simulink model "P414_1_model02"  (R2021a)
settings: Solver=VariableStepAuto  StartTime=0.0  StopTime=1  RelTol=1e-3
values from neighbouring files (symbols this model uses):
  crop__C = [0.01 0.001 0.01 0.01]    [params.mat]
  crop__N = [0 0 0 0 0 0 0 0]    [params.mat]
  crop__R = [0 0 0]    [params.mat]
  heater__T = 288    [params.mat]
  subtrate__N = [1e-06 1e-06 1e-06 1e-06 1e-06 1e-06 1e-06 1e-06]    [params.mat]
  Tmax = 296    [P414_1_script.m]    (also in params.mat)
  Tstart = 285.5    [P414_1_script.m]    (also in params.mat)
libraries: HORTISIM x15
settings Model: VariantFading=off  Creator=djoroya  LastModifiedBy=djoroya
settings SolverCC: MaxConsecutiveMinStep=2
settings HardwareCC: TargetBitPerLong=64  TargetBitPerPointer=64  TargetBitPerSizeT=64  TargetBitPerPtrDiffT=64  TargetLongLongMode=on  TargetIntDivRoundTo=Zero  TargetEndianess=LittleEndian  TargetWordSize=64  TargetHWDeviceType=MATLAB Host  ProdEqTarget=off
settings RTWCC: Description=Rapid Simulation Target  SystemTargetFile=rsim.tlc  TemplateMakefile=rsim_default_tmf
settings RSimTargetCC: TargetLangStandard=C99 (ISO)

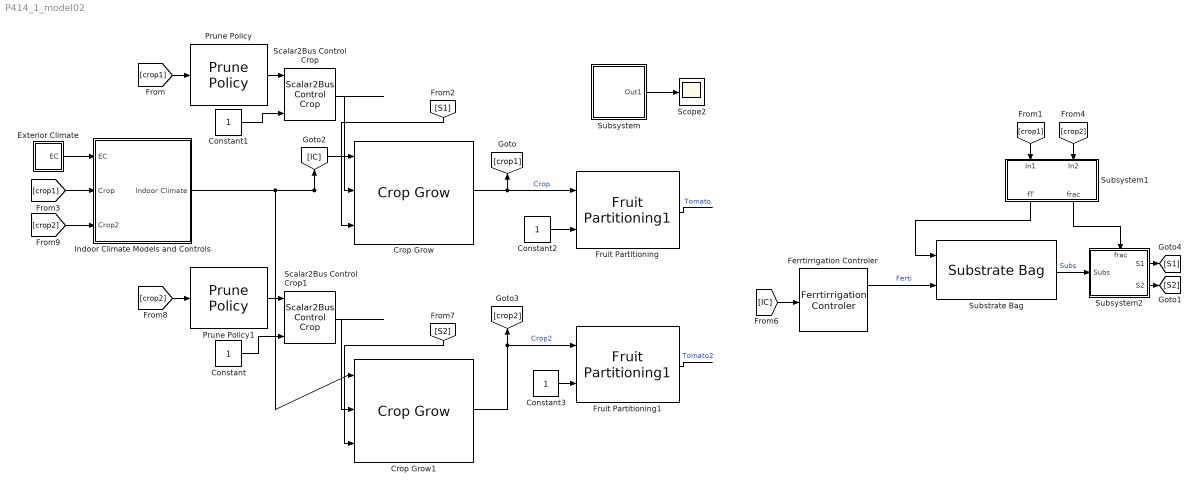
== system P414_1_model02 ==
  Constant{,1..3} (4 alike) : Constant
  Crop Grow : HORTISIM/Horticulture/Models/Crop Grow  Chi_nutrients=crop__Chi_nutrients  A_v=crop__A_v  plants_density=crop__plants_density  fraction_DM=crop__fraction_DM  min_water_capacity=crop__min_water_capacity  C_buf_max=crop__C_buf_max  T_v_start_fruit=crop__T_v_start_fruit  int_air_speed=crop__int_air_speed  b_N_uptake=crop__b_N_uptake  Tv=crop__Tv  C=crop__C  R=crop__R  Tsum=crop__Tsum  C_wv=crop__C_wv  N=crop__N  rg_fruit=crop__rg_fruit  c_fruit_m=crop__c_fruit_m  c_fruit_g=crop__c_fruit_g  rg_leaf=crop__rg_leaf  c_leaf_m=crop__c_leaf_m  c_leaf_g=crop__c_leaf_g  rg_stem=crop__rg_stem  c_stem_m=crop__c_stem_m  c_stem_g=crop__c_stem_g  VelocityAbsortion=crop__VelocityAbsortion  T_max_v=crop__T_max_v  s_max_T=crop__s_max_T  s_min_T=crop__s_min_T  s_buforg_buf=crop__s_buforg_buf  T_sum_end=crop__T_sum_end  T_max_v24=crop__T_max_v24  T_min_v24=crop__T_min_v24  s_min_T24=crop__s_min_T24  s_max_T24=crop__s_max_T24  T_min_v=crop__T_min_v
      settings: SourceProductName=Horti Simulator
  Crop Grow1 : HORTISIM/Horticulture/Models/Crop Grow  Chi_nutrients=crop__Chi_nutrients  A_v=crop__A_v  plants_density=crop__plants_density  fraction_DM=crop__fraction_DM  min_water_capacity=crop__min_water_capacity  C_buf_max=crop__C_buf_max  T_v_start_fruit=crop__T_v_start_fruit  int_air_speed=crop__int_air_speed  b_N_uptake=crop__b_N_uptake  Tv=crop__Tv  C=crop__C  R=crop__R  Tsum=crop__Tsum  C_wv=crop__C_wv  N=crop__N  rg_fruit=crop__rg_fruit  c_fruit_m=crop__c_fruit_m  c_fruit_g=crop__c_fruit_g  rg_leaf=crop__rg_leaf  c_leaf_m=crop__c_leaf_m  c_leaf_g=crop__c_leaf_g  rg_stem=crop__rg_stem  c_stem_m=crop__c_stem_m  c_stem_g=crop__c_stem_g  VelocityAbsortion=crop__VelocityAbsortion  T_max_v=crop__T_max_v  s_max_T=crop__s_max_T  s_min_T=crop__s_min_T  s_buforg_buf=crop__s_buforg_buf  T_sum_end=crop__T_sum_end  T_max_v24=crop__T_max_v24  T_min_v24=crop__T_min_v24  s_min_T24=crop__s_min_T24  s_max_T24=crop__s_max_T24  T_min_v=crop__T_min_v
      settings: SourceProductName=Horti Simulator
  Exterior Climate : Subsystem
  Ferrtirrigation Controler : HORTISIM/Horticulture/Controls/Ferrtirrigation  Controler  hour0=irrigation__hour0  IrrigationFlow=irrigation__IrrigationFlow  Xnutrients=irrigation__Xnutrients  percent_irrigation=irrigation__percent_irrigation  Irrigation_jules_to_hours=irrigation__Irrigation_jules_to_hours
      settings: SourceProductName=Horti Simulator
  Fruit Partitioning : HORTISIM/Horticulture/Models/Fruit Partitioning1  Cfruit0=tomato__Cfruit0
      settings: SourceProductName=Horti Simulator
  Fruit Partitioning1 : HORTISIM/Horticulture/Models/Fruit Partitioning1  Cfruit0=tomato__Cfruit0
      settings: SourceProductName=Horti Simulator
  Indoor Climate Models and Controls : Subsystem
  Prune Policy : HORTISIM/Horticulture/Controls/Prune Policy  SystemSampleTime=-1  VariantActivationTime=update diagram  Latency=0  AutoFrameSizeCalculation=off
      settings: SourceProductName=Horti Simulator
  Prune Policy1 : HORTISIM/Horticulture/Controls/Prune Policy  SystemSampleTime=-1  VariantActivationTime=update diagram  Latency=0  AutoFrameSizeCalculation=off
      settings: SourceProductName=Horti Simulator
  Scalar2Bus Control Crop : HORTISIM/Other  Functions/Scalar2Bus Control Crop  SystemSampleTime=-1  VariantActivationTime=update diagram  Latency=0  AutoFrameSizeCalculation=off
      settings: SourceProductName=Horti Simulator
  Scalar2Bus Control Crop1 : HORTISIM/Other  Functions/Scalar2Bus Control Crop  SystemSampleTime=-1  VariantActivationTime=update diagram  Latency=0  AutoFrameSizeCalculation=off
      settings: SourceProductName=Horti Simulator
  Scope2 : Scope
  Substrate Bag : HORTISIM/Horticulture/Models/Substrate Bag  Vmax_subs=subtrate__Vmax_subs  Vmin_subs=subtrate__Vmin_subs  Nmin_subs=subtrate__Nmin_subs  C_ws=subtrate__C_ws  N=subtrate__N  DraingeConst=subtrate__DraingeConst  sigma_max=subtrate__sigma_max  sigma_min=subtrate__sigma_min
      settings: SourceProductName=Horti Simulator
  Subsystem : Subsystem  mask{tinit=0.5, tend=0.8}
  Subsystem1 : Subsystem
  Subsystem2 : Subsystem
      settings: PortSchema="{\"entries\":[{\"content\":{\"sides\":[{\"content\":{\"connectorIds\":[\"In1\"]},\"type\":\"ConnectorPlacement.EquallySpacedRectSide\",\"uuid\":\"526c2ba0-7984-4a67-b75e-815cf79b4473\"},{\"content\":{\"connectorIds\":[\"Out1\",\"Out2\"],\"side\":\"RIGHT\"},\"type\":\"ConnectorPlacement.EquallySpacedRectSide\",\"uuid\":\"1f428ce7-4be7-4b4c-9b6b-ebbf12a2ebe7\"},{\"content\":{\"connectorIds\":[\"In2\"],\"side\":\"TOP\"},\"type\":\"ConnectorPlacement.EquallySpacedRectSide\",\"uuid\":\"5866ee80-50d2-4205-943e-212db577b0a0\"}]},\"type\":\"ConnectorPlacement.EquallySpacedConnector\",\"uuid\":\"0f7aadc1-005b-462a-894f-416c66164dac\"}],\"packageUris\":[\"http://schema.mathworks.com/mf0/Connector/R2020b\"],\"version\":\"1.0\"}"
  wires:
  Exterior Climate/1(EC) -> Indoor Climate Models and Controls/1(EC)
  Indoor Climate Models and Controls/1(Indoor Climate) -> Crop Grow1/1, [IC], Crop Grow/1
  Crop Grow/1 -> [crop1], Fruit Partitioning/1  "Crop"
  Ferrtirrigation Controler/1 -> Substrate Bag/2  "Ferti"
  Scalar2Bus Control Crop/1 -> Crop Grow/2
  Prune Policy/1 -> Scalar2Bus Control Crop/1
  [crop1] -> Prune Policy/1
  [S1] -> Crop Grow/3
  [crop1] -> Indoor Climate Models and Controls/2(Crop)
  Fruit Partitioning/1 -> ?  "Tomato"
  [IC] -> Ferrtirrigation Controler/1
  Crop Grow1/1 -> [crop2], Fruit Partitioning1/1  "Crop2"
  Fruit Partitioning1/1 -> ?  "Tomato2"
  Subsystem/1(Out1) -> Scope2/1
  [S2] -> Crop Grow1/3
  [crop2] -> Prune Policy1/1
  Scalar2Bus Control Crop1/1 -> Crop Grow1/2
  Prune Policy1/1 -> Scalar2Bus Control Crop1/1
  Constant/1 -> Scalar2Bus Control Crop1/4
  Constant1/1 -> Scalar2Bus Control Crop/4
  Constant2/1 -> Fruit Partitioning/2
  Constant3/1 -> Fruit Partitioning1/2
  [crop2] -> Indoor Climate Models and Controls/3(Crop2)
  [crop1] -> Subsystem1/1(In1)
  [crop2] -> Subsystem1/2(In2)
  Subsystem1/1(fT) -> Substrate Bag/1
  Substrate Bag/1 -> Subsystem2/1(Subs)  "Subs"
  Subsystem1/2(frac) -> Subsystem2/2(frac)
  Subsystem2/2(S2) -> [S2]
  Subsystem2/1(S1) -> [S1]

== system P414_1_model02/Exterior Climate ==
  Demux : Demux
  From Workspace : FromWorkspace  VariableName=EC
  Scalar2Bus Exterior Climate : Subsystem
  EC : Outport
  wires:
  Demux/3 -> Scalar2Bus Exterior Climate/3(Wind)
  Demux/2 -> Scalar2Bus Exterior Climate/2(Radiation)
  Scalar2Bus Exterior Climate/1(EC) -> EC/1
  Demux/1 -> Scalar2Bus Exterior Climate/1(Temperature)
  Demux/4 -> Scalar2Bus Exterior Climate/4(Humidity)
  From Workspace/1 -> Demux/1

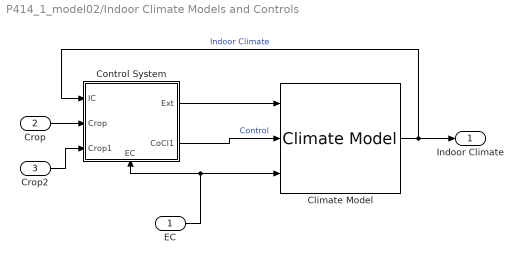
== system P414_1_model02/Indoor Climate Models and Controls ==
  EC : Inport
  Crop : Inport  Port=2
  Crop2 : Inport  Port=3
  Climate Model : HORTISIM/Climate/Models/Climate Model  hour0=clima__hour0  G0=clima__G0  T0=clima__T0  H=clima__H  A_f=clima__A_f  A_c=clima__A_c  minWindows=clima__minWindows  lam_s=clima__lam_s  c_s=clima__c_s  l_s=clima__l_s  rhod_s=clima__rhod_s  int_air_speed=clima__int_air_speed  alpha_i=clima__alpha_i  alpha_c=clima__alpha_c  tau_c=clima__tau_c  alpha_f=clima__alpha_f  d_c=clima__d_c  cd_c=clima__cd_c  T_ss=clima__T_ss
      settings: SourceProductName=Horti Simulator
  Control System : Subsystem
      settings: PortSchema="{\"entries\":[{\"content\":{\"sides\":[{\"content\":{\"connectorIds\":[\"In1\",\"In2\",\"In3\"]},\"type\":\"ConnectorPlacement.EquallySpacedRectSide\",\"uuid\":\"7d0146e2-a53b-49ab-a7f4-04cd7ef00b9a\"},{\"content\":{\"connectorIds\":[\"Out1\",\"Out2\"],\"side\":\"RIGHT\"},\"type\":\"ConnectorPlacement.EquallySpacedRectSide\",\"uuid\":\"fee587e2-4b5c-4140-8904-07609d427593\"},{\"content\":{\"connectorIds\":[],\"side\":\"TOP\"},\"type\":\"ConnectorPlacement.EquallySpacedRectSide\",\"uuid\":\"52e767bc-1595-40ac-996f-44c9eedd0a08\"},{\"content\":{\"connectorIds\":[\"In4\"],\"side\":\"BOTTOM\"},\"type\":\"ConnectorPlacement.EquallySpacedRectSide\",\"uuid\":\"c629db5c-cfe6-4bd1-aeb9-7fba46dde396\"}]},\"type\":\"ConnectorPlacement.EquallySpacedConnector\",\"uuid\":\"268fde01-3c08-4d62-bfbb-fc94284c5cdd\"}],\"packageUris\":[\"http://schema.mathworks.com/mf0/Connector/R2020b\"],\"version\":\"1.0\"}"
  Indoor Climate : Outport
  wires:
  Climate Model/1 -> Indoor Climate/1, Control System/1(IC)  "Indoor Climate"
  Control System/2(CoCl1) -> Climate Model/2  "Control"
  Control System/1(Ext) -> Climate Model/1
  EC/1 -> Control System/4(EC), Climate Model/3
  Crop/1 -> Control System/2(Crop)
  Crop2/1 -> Control System/3(Crop1)

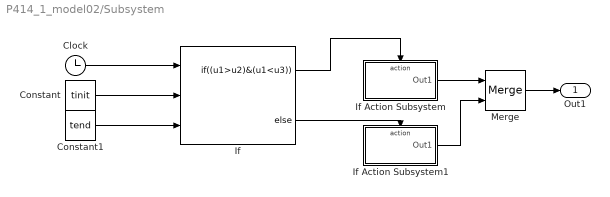
== system P414_1_model02/Subsystem ==
  Clock : Clock
  Constant : Constant  Value=tinit
  Constant1 : Constant  Value=tend
  If : If  NumInputs=3  IfExpression=(u1>u2)&(u1<u3)
  If Action Subsystem : Subsystem  TreatAsAtomicUnit=on
  If Action Subsystem1 : Subsystem  TreatAsAtomicUnit=on
  Merge : Merge
  Out1 : Outport
  wires:
  Clock/1 -> If/1
  Constant/1 -> If/2
  Constant1/1 -> If/3
  If/1 -> If Action Subsystem/Action
  If/2 -> If Action Subsystem1/Action
  If Action Subsystem/1(Out1) -> Merge/1
  If Action Subsystem1/1(Out1) -> Merge/2
  Merge/1 -> Out1/1

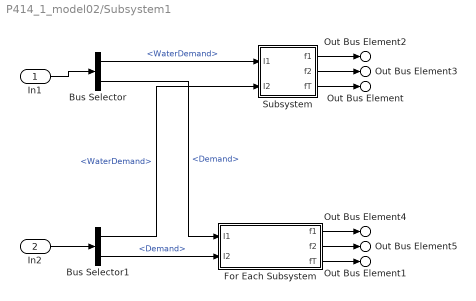
== system P414_1_model02/Subsystem1 ==
  In1 : Inport
  In2 : Inport  Port=2
  Bus Selector : BusSelector  OutputSignals=Water.WaterFlows.WaterDemand,Nutrients.Demand
  Bus Selector1 : BusSelector  OutputSignals=Water.WaterFlows.WaterDemand,Nutrients.Demand
  For Each Subsystem : Subsystem  TreatAsAtomicUnit=on
  Subsystem : Subsystem
  Out Bus Element1 : Outport  PortName=fT  Element=Nutrients.Demand
  Out Bus Element : Outport  PortName=fT  Element=Water.WaterFlows.WaterDemand
  Out Bus Element2 : Outport  Port=2  PortName=frac  Element=water.f1
  Out Bus Element3 : Outport  Port=2  PortName=frac  Element=water.f2
  Out Bus Element4 : Outport  Port=2  PortName=frac  Element=nutrients.f1
  Out Bus Element5 : Outport  Port=2  PortName=frac  Element=nutrients.f2
  wires:
  In1/1 -> Bus Selector/1
  In2/1 -> Bus Selector1/1
  Bus Selector1/1 -> Subsystem/2(I2)  "<WaterDemand>"
  Bus Selector/1 -> Subsystem/1(I1)  "<WaterDemand>"
  Subsystem/3(fT) -> Out Bus Element/1
  Subsystem/1(f1) -> Out Bus Element2/1
  Subsystem/2(f2) -> Out Bus Element3/1
  Bus Selector/2 -> For Each Subsystem/1(I1)  "<Demand>"
  Bus Selector1/2 -> For Each Subsystem/2(I2)  "<Demand>"
  For Each Subsystem/3(fT) -> Out Bus Element1/1
  For Each Subsystem/2(f2) -> Out Bus Element5/1
  For Each Subsystem/1(f1) -> Out Bus Element4/1

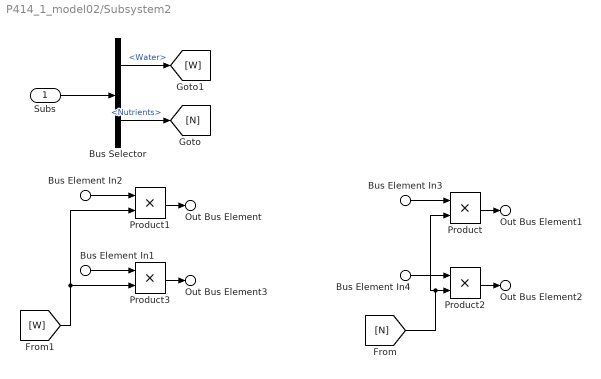
== system P414_1_model02/Subsystem2 ==
  Subs : Inport
  Bus Element In2 : Inport  Port=2  PortName=frac  Element=water.f1
  Bus Element In1 : Inport  Port=2  PortName=frac  Element=water.f2
  Bus Element In3 : Inport  Port=2  PortName=frac  Element=nutrients.f1
  Bus Element In4 : Inport  Port=2  PortName=frac  Element=nutrients.f2
  Bus Selector : BusSelector  OutputSignals=Uptake.Water,Uptake.Nutrients
  Product{,1..3} (4 alike) : Product
  Out Bus Element : Outport  PortName=S1  Element=Uptake.Water
  Out Bus Element1 : Outport  PortName=S1  Element=Uptake.Nutrients
  Out Bus Element3 : Outport  Port=2  PortName=S2  Element=Uptake.Water
  Out Bus Element2 : Outport  Port=2  PortName=S2  Element=Uptake.Nutrients
  wires:
  Subs/1 -> Bus Selector/1
  Bus Selector/1 -> [W]  "<Water>"
  Bus Selector/2 -> [N]  "<Nutrients>"
  Bus Element In3/1 -> Product/1
  Bus Element In2/1 -> Product1/1
  Bus Element In4/1 -> Product2/1
  [N] -> Product/2, Product2/2
  Bus Element In1/1 -> Product3/1
  [W] -> Product3/2, Product1/2
  Product1/1 -> Out Bus Element/1
  Product3/1 -> Out Bus Element3/1
  Product/1 -> Out Bus Element1/1
  Product2/1 -> Out Bus Element2/1

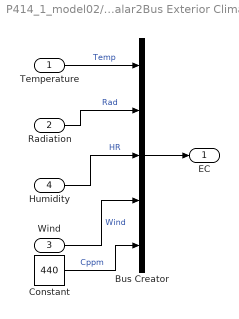
== system P414_1_model02/Exterior Climate/Scalar2Bus Exterior Climate ==
  Temperature : Inport
  Radiation : Inport  Port=2
  Wind : Inport  Port=3
  Humidity : Inport  Port=4
  Bus Creator : BusCreator  Inputs=5
  Constant : Constant  Value=440
  EC : Outport
  wires:
  Humidity/1 -> Bus Creator/3  "HR"
  Wind/1 -> Bus Creator/4  "Wind"
  Temperature/1 -> Bus Creator/1  "Temp"
  Bus Creator/1 -> EC/1
  Radiation/1 -> Bus Creator/2  "Rad"
  Constant/1 -> Bus Creator/5  "Cppm"

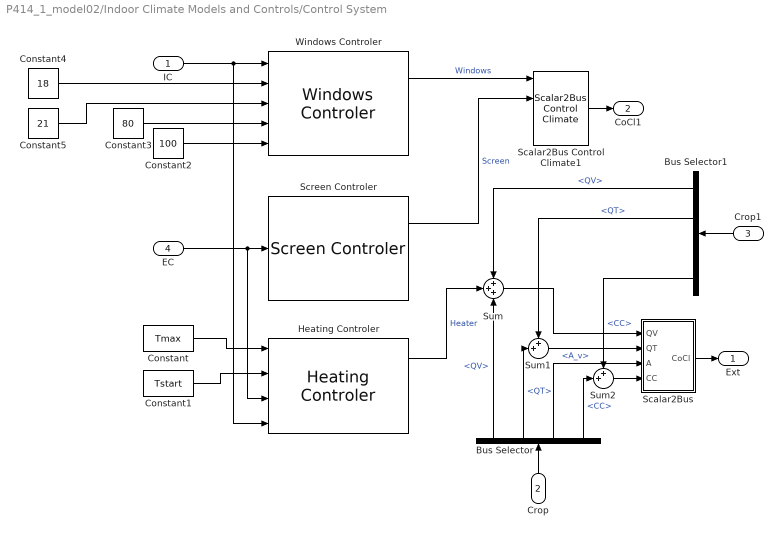
== system P414_1_model02/Indoor Climate Models and Controls/Control System ==
  IC : Inport
  Crop : Inport  Port=2
  Crop1 : Inport  Port=3
  EC : Inport  Port=4
  Bus Selector : BusSelector  OutputSignals=HeatVars.QV,HeatVars.QT,A_v,CC
  Bus Selector1 : BusSelector  OutputSignals=HeatVars.QV,HeatVars.QT,A_v,CC
  Constant : Constant  Value=Tmax
  Constant1 : Constant  Value=Tstart
  Constant2 : Constant  Value=100
  Constant3 : Constant  Value=80
  Constant4 : Constant  Value=18
  Constant5 : Constant  Value=21
  Heating Controler : HORTISIM/Climate/Controls/Heating Controler  T=heater__T  power=heater__power  A_e=heater__A_e  A_i=heater__A_i  c=heater__c
      settings: SourceProductName=Horti Simulator
  "Scalar2Bus " : Subsystem
  Scalar2Bus Control Climate1 : HORTISIM/Other  Functions/Scalar2Bus  Control Climate  SystemSampleTime=-1  VariantActivationTime=update diagram  Latency=0  AutoFrameSizeCalculation=off
      settings: SourceProductName=Horti Simulator
  Screen Controler : HORTISIM/Climate/Controls/Screen Controler  Radthreshold=screen__Radthreshold  velocity=screen__velocity  Power=screen__Power  gamma_max=screen__gamma_max  beta=screen__beta
      settings: SourceProductName=Horti Simulator
  Sum : Sum  Inputs=+++
  Sum1 : Sum  Inputs=++|
  Sum2 : Sum  Inputs=++|
  Windows Controler : HORTISIM/Climate/Controls/Windows Controler  Power=windows__Power  max_night=windows__max_night  tau=windows__tau  RadThreshold=windows__RadThreshold  AR=windows__AR
      settings: SourceProductName=Horti Simulator
  Ext : Outport
  CoCl1 : Outport  Port=2
  wires:
  EC/1 -> Heating Controler/3, Screen Controler/1
  "Scalar2Bus "/1(CoCl) -> Ext/1
  Constant1/1 -> Heating Controler/2
  Constant/1 -> Heating Controler/1
  Windows Controler/1 -> Scalar2Bus Control Climate1/1  "Windows"
  Scalar2Bus Control Climate1/1 -> CoCl1/1
  Screen Controler/1 -> Scalar2Bus Control Climate1/2  "Screen"
  IC/1 -> Heating Controler/4, Windows Controler/1
  Constant2/1 -> Windows Controler/5
  Constant3/1 -> Windows Controler/4
  Constant4/1 -> Windows Controler/2
  Constant5/1 -> Windows Controler/3
  Crop/1 -> Bus Selector/1
  Sum/1 -> "Scalar2Bus "/1(QV)
  Bus Selector/3 -> "Scalar2Bus "/3(A)  "<A_v>"
  Crop1/1 -> Bus Selector1/1
  Bus Selector/1 -> Sum/3  "<QV>"
  Heating Controler/1 -> Sum/2  "Heater"
  Bus Selector1/1 -> Sum/1  "<QV>"
  Sum1/1 -> "Scalar2Bus "/2(QT)
  Bus Selector/2 -> Sum1/2  "<QT>"
  Bus Selector1/2 -> Sum1/1  "<QT>"
  Sum2/1 -> "Scalar2Bus "/4(CC)
  Bus Selector/4 -> Sum2/2  "<CC>"
  Bus Selector1/4 -> Sum2/1  "<CC>"

== system P414_1_model02/Subsystem/If Action Subsystem ==
  Action Port : ActionPort  ActionPortLabel=if((u1>u2)&(u1<u3))
  Constant : Constant
  Out1 : Outport
  wires:
  Constant/1 -> Out1/1

== system P414_1_model02/Subsystem/If Action Subsystem1 ==
  Action Port : ActionPort  ActionPortLabel=else
  Constant : Constant  Value=0
  Out1 : Outport
  wires:
  Constant/1 -> Out1/1

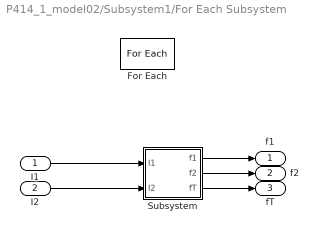
== system P414_1_model02/Subsystem1/For Each Subsystem ==
  I1 : Inport  Partition=on  PartitionDimension=1  PartitionWidth=1  PartitionOffset=0
  I2 : Inport  Port=2  Partition=on  PartitionDimension=1  PartitionWidth=1  PartitionOffset=0
  For Each : ForEach  DisableCoverage=on
  Subsystem : Subsystem
  f1 : Outport  ConcatenationDimension=1
  f2 : Outport  Port=2  ConcatenationDimension=1
  fT : Outport  Port=3  ConcatenationDimension=1
  wires:
  I2/1 -> Subsystem/2(I2)
  I1/1 -> Subsystem/1(I1)
  Subsystem/3(fT) -> fT/1
  Subsystem/2(f2) -> f2/1
  Subsystem/1(f1) -> f1/1

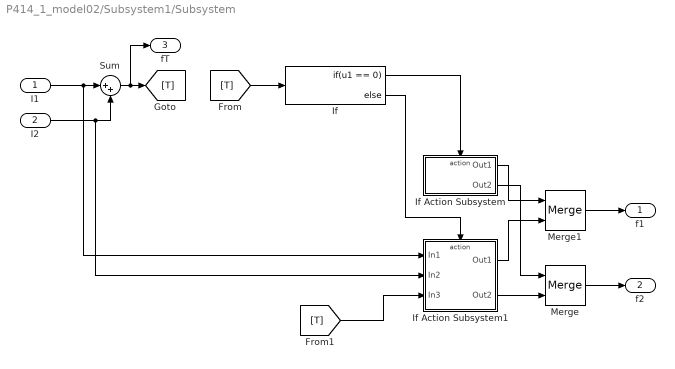
== system P414_1_model02/Subsystem1/Subsystem ==
  I1 : Inport
  I2 : Inport  Port=2
  If : If  IfExpression=u1 == 0
  If Action Subsystem : Subsystem  TreatAsAtomicUnit=on
  If Action Subsystem1 : Subsystem  TreatAsAtomicUnit=on
  Merge : Merge
  Merge1 : Merge
  Sum : Sum  Inputs=|++
  f1 : Outport
  f2 : Outport  Port=2
  fT : Outport  Port=3
  wires:
  I1/1 -> If Action Subsystem1/1(In1), Sum/1
  I2/1 -> If Action Subsystem1/2(In2), Sum/2
  Sum/1 -> fT/1, [T]
  [T] -> If/1
  If/1 -> If Action Subsystem/Action
  If/2 -> If Action Subsystem1/Action
  [T] -> If Action Subsystem1/3(In3)
  If Action Subsystem/2(Out2) -> Merge/1
  If Action Subsystem1/2(Out2) -> Merge/2
  Merge/1 -> f2/1
  Merge1/1 -> f1/1
  If Action Subsystem1/1(Out1) -> Merge1/2
  If Action Subsystem/1(Out1) -> Merge1/1

== system P414_1_model02/Indoor Climate Models and Controls/Control System/Scalar2Bus  ==
  QV : Inport
  QT : Inport  Port=2
  A : Inport  Port=3
  CC : Inport  Port=4
  Bus Creator : BusCreator  Inputs=4
  CoCl : Outport
  wires:
  A/1 -> Bus Creator/3  "A"
  CC/1 -> Bus Creator/4  "CC"
  QV/1 -> Bus Creator/1  "QV"
  Bus Creator/1 -> CoCl/1
  QT/1 -> Bus Creator/2  "QT"

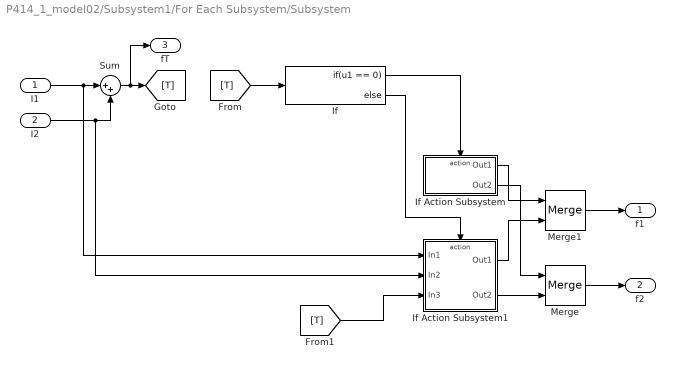
== system P414_1_model02/Subsystem1/For Each Subsystem/Subsystem ==
  I1 : Inport
  I2 : Inport  Port=2
  If : If  IfExpression=u1 == 0
  If Action Subsystem : Subsystem  TreatAsAtomicUnit=on
  If Action Subsystem1 : Subsystem  TreatAsAtomicUnit=on
  Merge : Merge
  Merge1 : Merge
  Sum : Sum  Inputs=|++
  f1 : Outport
  f2 : Outport  Port=2
  fT : Outport  Port=3
  wires:
  I1/1 -> If Action Subsystem1/1(In1), Sum/1
  I2/1 -> If Action Subsystem1/2(In2), Sum/2
  Sum/1 -> fT/1, [T]
  [T] -> If/1
  If/1 -> If Action Subsystem/Action
  If/2 -> If Action Subsystem1/Action
  [T] -> If Action Subsystem1/3(In3)
  If Action Subsystem/2(Out2) -> Merge/1
  If Action Subsystem1/2(Out2) -> Merge/2
  Merge/1 -> f2/1
  Merge1/1 -> f1/1
  If Action Subsystem1/1(Out1) -> Merge1/2
  If Action Subsystem/1(Out1) -> Merge1/1

== system P414_1_model02/Subsystem1/Subsystem/If Action Subsystem ==
  Action Port : ActionPort  ActionPortLabel=if(u1 == 0)
  Constant : Constant  Value=0
  Constant1 : Constant  Value=0
  Out1 : Outport
  Out2 : Outport  Port=2
  wires:
  Constant/1 -> Out1/1
  Constant1/1 -> Out2/1

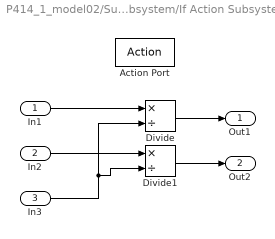
== system P414_1_model02/Subsystem1/Subsystem/If Action Subsystem1 ==
  In1 : Inport
  In2 : Inport  Port=2
  In3 : Inport  Port=3
  Action Port : ActionPort  ActionPortLabel=else
  Divide : Product  Inputs=*/
  Divide1 : Product  Inputs=*/
  Out1 : Outport
  Out2 : Outport  Port=2
  wires:
  In1/1 -> Divide/1
  In2/1 -> Divide1/1
  In3/1 -> Divide1/2, Divide/2
  Divide/1 -> Out1/1
  Divide1/1 -> Out2/1

== system P414_1_model02/Subsystem1/For Each Subsystem/Subsystem/If Action Subsystem ==
  Action Port : ActionPort  ActionPortLabel=if(u1 == 0)
  Constant : Constant  Value=0
  Constant1 : Constant  Value=0
  Out1 : Outport
  Out2 : Outport  Port=2
  wires:
  Constant/1 -> Out1/1
  Constant1/1 -> Out2/1

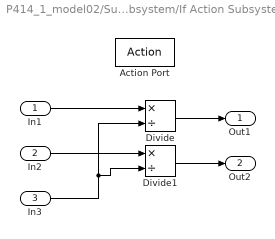
== system P414_1_model02/Subsystem1/For Each Subsystem/Subsystem/If Action Subsystem1 ==
  In1 : Inport
  In2 : Inport  Port=2
  In3 : Inport  Port=3
  Action Port : ActionPort  ActionPortLabel=else
  Divide : Product  Inputs=*/
  Divide1 : Product  Inputs=*/
  Out1 : Outport
  Out2 : Outport  Port=2
  wires:
  In1/1 -> Divide/1
  In2/1 -> Divide1/1
  In3/1 -> Divide1/2, Divide/2
  Divide/1 -> Out1/1
  Divide1/1 -> Out2/1
